simulink library "Custom_Lib"  (R2020b)
settings: Solver=VariableStepAuto  StartTime=0.0  StopTime=10.0  RelTol=1e-3
libraries: dspxfrm3 x2, simulink x1
settings Model: Creator=AlexKurash  LastModifiedBy=AlexKurash

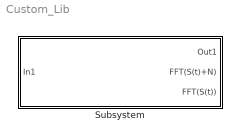
== system Custom_Lib ==
  Subsystem : Subsystem  mask(Fourier Filtration){FFT_Length=1024, ThrValue=150}
      mask prompts: FFT_Length "FFT Length (число точек БПФ):"; ThrValue "Thresshold Value (Пороговое Значение)"
      mask help:
      | ENG: This block performs bandpass interference rejection based on the fast Fourier transform algorithm, the rejection is performed by comparing the components with the threshold level, and zeroing the components that exceed the specified threshold.
      |
      | The threshold level can be set based on graphically visualized FFT results that can be obtained from the debug ports.
      | ----------------------------------------
      | RUS: Данный блок осуществляет режекцию полосовых помех на основании алгоритма быстрого преобразования фурье, режекция осуществляется путем сравнения компонент с пороговым уровнем, и обнулением компоненты превышающих заданный порог.
      |
      | Настройку порогового уровня можно осуществить на основании графически-визуализированных результатов FFT , которые могут быть получены с портов отладки
      | ----------------------------------------
      mask Display:
      | disp ('FFT filtration')
      | port_label('input', 1, 'S(t)+N')
      | port_label('output', 1, 'S(t)')
      | port_label('output', 2, 'FFT(S(t)+N)')
      | port_label('output', 3, 'FFT(S(t))')

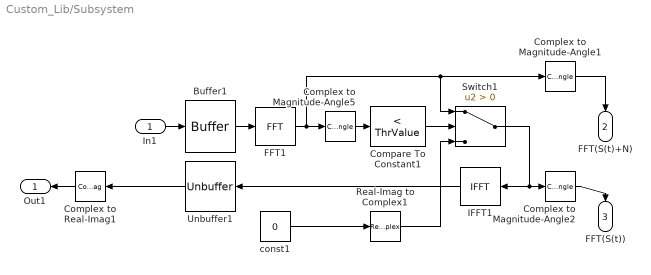
== system Custom_Lib/Subsystem ==
  In1 : Inport
  Buffer1 : Buffer  N=FFT_Length  OutputFrames=off
  Compare To Constant1 : simulink/Logic and Bit Operations/Compare To Constant  relop=<  const=ThrValue  OutDataTypeStr=boolean
  Complex to Magnitude-Angle1 : ComplexToMagnitudeAngle  Output=Magnitude
  Complex to Magnitude-Angle2 : ComplexToMagnitudeAngle  Output=Magnitude
  Complex to Magnitude-Angle5 : ComplexToMagnitudeAngle  Output=Magnitude
  Complex to Real-Imag1 : ComplexToRealImag  Output=Real
  FFT1 : dspxfrm3/FFT  FFTImplementation=Auto  CompMethod=Table lookup  TableOpt=NEW  TableOptActive=Speed  BitRevOrder=off  Normalize=off  InheritFFTLength=on  FFTLength=FFT_Length  WrapInput=on  roundingMode=Floor  overflowMode=off  firstCoeffDataTypeStr=Inherit: Same word length as input  firstCoeffLastDataTypeStr=Inherit: Same word length as input  outputMin=[]  outputMax=[]
  IFFT1 : dspxfrm3/IFFT  FFTImplementation=Auto  CompMethod=Table lookup  TableOpt=NEW  TableOptActive=Speed  BitRevOrder=off  cs_in=off  Normalize=on  InheritFFTLength=on  FFTLength=FFT_Length  WrapInput=on  mode=Complex  outSamplingMode=Sample based  roundingMode=Floor  overflowMode=off  firstCoeffDataTypeStr=Inherit: Same word length as input  firstCoeffLastDataTypeStr=Inherit: Same word length as input  outputMin=[]  outputMax=[]
  Real-Imag to Complex1 : RealImagToComplex  Input=Real
  Switch1 : Switch  Criteria=u2 > Threshold
  Unbuffer1 : Unbuffer
  const1 : Constant  Value=0  OutDataTypeStr=Inherit: Inherit via back propagation
  Out1 : Outport
  FFT(S(t)+N) : Outport  Port=2
  FFT(S(t)) : Outport  Port=3
  wires:
  Real-Imag to Complex1/1 -> Switch1/3
  FFT1/1 -> Complex to Magnitude-Angle5/1, Complex to Magnitude-Angle1/1, Switch1/1
  Complex to Magnitude-Angle2/1 -> FFT(S(t))/1
  Complex to Magnitude-Angle1/1 -> FFT(S(t)+N)/1
  Complex to Real-Imag1/1 -> Out1/1
  Unbuffer1/1 -> Complex to Real-Imag1/1
  Compare To Constant1/1 -> Switch1/2
  Complex to Magnitude-Angle5/1 -> Compare To Constant1/1
  const1/1 -> Real-Imag to Complex1/1
  IFFT1/1 -> Unbuffer1/1
  In1/1 -> Buffer1/1
  Switch1/1 -> IFFT1/1, Complex to Magnitude-Angle2/1
  Buffer1/1 -> FFT1/1
